simulink model "gait_player_right_leg"  (R2015b)
settings: Solver=FixedStepDiscrete  StartTime=0.0  StopTime=inf  FixedStep=.001  RelTol=1e-3
libraries: xpcethercatlib x19, slrtlib x7
settings Model: SimulationMode=external  Creator=rtheyyun  LastModifiedBy=tech
settings SolverCC: EnableConcurrentExecution=on  ConcurrentTasks=on
settings DataIOCC: SaveFinalState=on  SaveFormat=StructureWithTime  SignalLoggingSaveFormat=ModelDataLogs  InspectSignalLogs=on
settings OptimizationCC: BlockReduction=off  OptimizeBlockIOStorage=off  BufferReuse=off  GlobalBufferReuse=off  ExpressionFolding=off  ExpressionDepthLimit=2147483647  LocalBlockOutputs=off
settings DebuggingCC: ReadBeforeWriteMsg=DisableAll  WriteAfterWriteMsg=DisableAll  WriteAfterReadMsg=DisableAll  UnderspecifiedInitializationDetection=Classic  MergeDetectMultiDrivingBlocksExec=none  SolverPrmCheckMsg=warning  InheritedTsInSrcMsg=none  FcnCallInpInsideContextMsg=UseLocalSettings  StateNameClashWarn=warning
settings HardwareCC: ProdBitPerPointer=32  ProdLargestAtomicFloat=None  ProdWordSize=32  ProdLongLongMode=on  ProdHWDeviceType=Generic->32-bit x86 compatible
settings RTWCC: SystemTargetFile=slrt.tlc  TemplateMakefile=slrt_default_tmf  Description=Simulink Real-Time  RTWVerbose=off  RTWCompilerOptimization=on
settings SimulinkRealTimeCC: GeneratePreprocessorConditionals=Disable all  xPCisModelTimeout=off  xPCModelTimeoutSecs=20  xPCConcurrentTasks=on
settings ConfigComp: CovModelRefEnable=Off  CovSFcnEnable=off

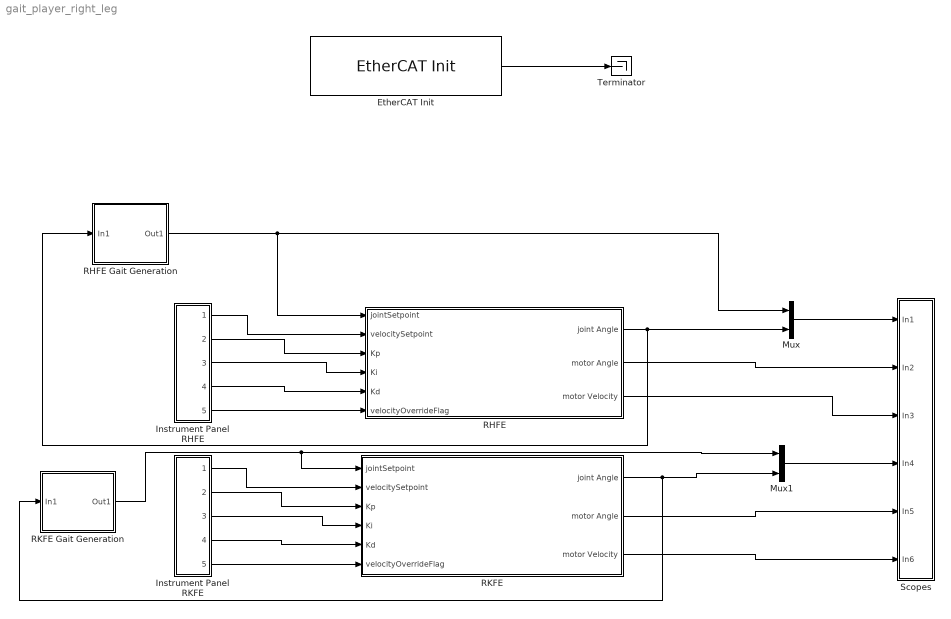
== system gait_player_right_leg ==
  "EtherCAT Init " : xpcethercatlib/EtherCAT Init   Priority=0  config_file=C:\Software\Simulink Realtime\Pre-recorded Gait\gait_player.xml  device_id=0  pci_bus=2  pci_slot=0  dctuning=0  enaDebug=off  enaDC=on  errLink=off  masterDbg=off  stateChgDbg=off  baseClock=off  masterCfg=off  logFile='c:\dbglog.txt'  sample_time=0.001000
  Instrument Panel RHFE : Subsystem
  Instrument Panel RKFE : Subsystem
  Mux : Mux  Inputs=2
  Mux1 : Mux  Inputs=2
  RHFE : Subsystem
  RHFE Gait Generation : Subsystem
  RKFE : Subsystem
  RKFE Gait Generation : Subsystem
  Scopes : Subsystem
  Terminator : Terminator
  wires:
  "EtherCAT Init "/1 -> Terminator/1
  Instrument Panel RHFE/1(Out2) -> RHFE/2("velocitySetpoint ")
  Instrument Panel RHFE/2(Out3) -> RHFE/3(Kp)
  Instrument Panel RHFE/3(Out4) -> RHFE/4(Ki)
  Instrument Panel RHFE/4(Out5) -> RHFE/5(Kd)
  Instrument Panel RHFE/5(Out6) -> RHFE/6(velocityOverrideFlag)
  Instrument Panel RKFE/1(Out2) -> RKFE/2("velocitySetpoint ")
  Instrument Panel RKFE/2(Out3) -> RKFE/3(Kp)
  Instrument Panel RKFE/3(Out4) -> RKFE/4(Ki)
  Instrument Panel RKFE/4(Out5) -> RKFE/5(Kd)
  Instrument Panel RKFE/5(Out6) -> RKFE/6(velocityOverrideFlag)
  RHFE/1(joint Angle) -> RHFE Gait Generation/1(In1), Mux/2
  RHFE/2(motor Angle) -> Scopes/2(In2)
  RHFE/3(motor Velocity) -> Scopes/3(In3)
  RKFE/1(joint Angle) -> RKFE Gait Generation/1(In1), Mux1/2
  RKFE/2(motor Angle) -> Scopes/5(In5)
  RKFE/3(motor Velocity) -> Scopes/6(In6)
  Mux/1 -> Scopes/1(In1)
  RHFE Gait Generation/1(Out1) -> RHFE/1(jointSetpoint), Mux/1
  Mux1/1 -> Scopes/4(In4)
  RKFE Gait Generation/1(Out1) -> RKFE/1(jointSetpoint), Mux1/1

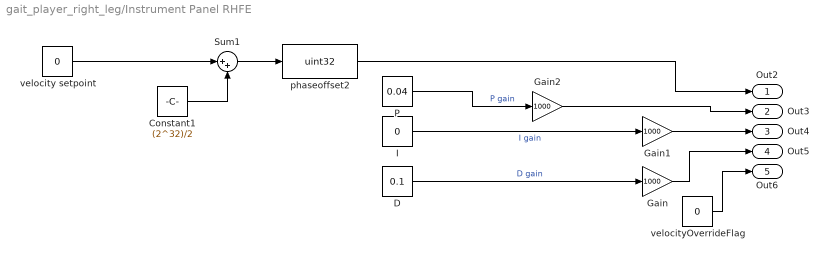
== system gait_player_right_leg/Instrument Panel RHFE ==
  Constant1 : Constant  Value=(2^32)/2
  D : Constant  Value=0.1  OutDataTypeStr=single
  Gain : Gain  Gain=1000  OutDataTypeStr=uint32
  Gain1 : Gain  Gain=1000  OutDataTypeStr=uint32
  Gain2 : Gain  Gain=1000  OutDataTypeStr=uint32
  I : Constant  Value=0  OutDataTypeStr=single
  P : Constant  Value=0.04  OutDataTypeStr=single
  Sum1 : Sum  Inputs=|++
  phaseoffset2 : DataTypeConversion  OutDataTypeStr=uint32
  velocity setpoint : Constant  Value=0  OutDataTypeStr=int16
  velocityOverrideFlag : Constant  Value=0  OutDataTypeStr=uint32
  Out2 : Outport
  Out3 : Outport  Port=2
  Out4 : Outport  Port=3
  Out5 : Outport  Port=4
  Out6 : Outport  Port=5
  wires:
  velocityOverrideFlag/1 -> Out6/1
  Gain2/1 -> Out3/1
  Constant1/1 -> Sum1/2
  Sum1/1 -> phaseoffset2/1
  velocity setpoint/1 -> Sum1/1
  phaseoffset2/1 -> Out2/1
  Gain1/1 -> Out4/1
  Gain/1 -> Out5/1
  I/1 -> Gain1/1  "I gain"
  D/1 -> Gain/1  "D gain"
  P/1 -> Gain2/1  "P gain"

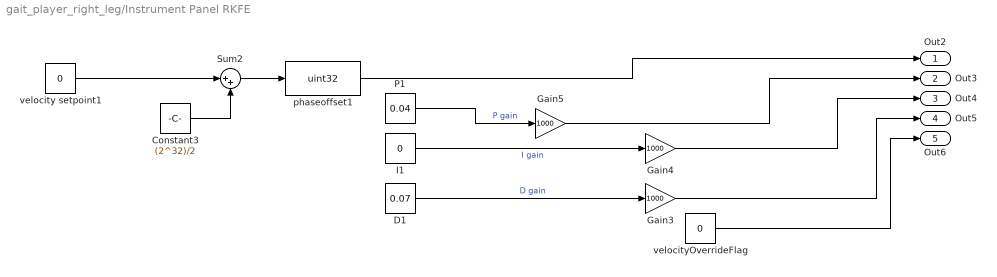
== system gait_player_right_leg/Instrument Panel RKFE ==
  Constant3 : Constant  Value=(2^32)/2
  D1 : Constant  Value=0.07  OutDataTypeStr=single
  Gain3 : Gain  Gain=1000  OutDataTypeStr=uint32
  Gain4 : Gain  Gain=1000  OutDataTypeStr=uint32
  Gain5 : Gain  Gain=1000  OutDataTypeStr=uint32
  I1 : Constant  Value=0  OutDataTypeStr=single
  P1 : Constant  Value=0.04  OutDataTypeStr=single
  Sum2 : Sum  Inputs=|++
  phaseoffset1 : DataTypeConversion  OutDataTypeStr=uint32
  velocity setpoint1 : Constant  Value=0  OutDataTypeStr=int16
  velocityOverrideFlag : Constant  Value=0  OutDataTypeStr=uint32
  Out2 : Outport
  Out3 : Outport  Port=2
  Out4 : Outport  Port=3
  Out5 : Outport  Port=4
  Out6 : Outport  Port=5
  wires:
  P1/1 -> Gain5/1  "P gain"
  Constant3/1 -> Sum2/2
  phaseoffset1/1 -> Out2/1
  Gain4/1 -> Out4/1
  Gain5/1 -> Out3/1
  I1/1 -> Gain4/1  "I gain"
  D1/1 -> Gain3/1  "D gain"
  Gain3/1 -> Out5/1
  velocityOverrideFlag/1 -> Out6/1
  velocity setpoint1/1 -> Sum2/1
  Sum2/1 -> phaseoffset1/1

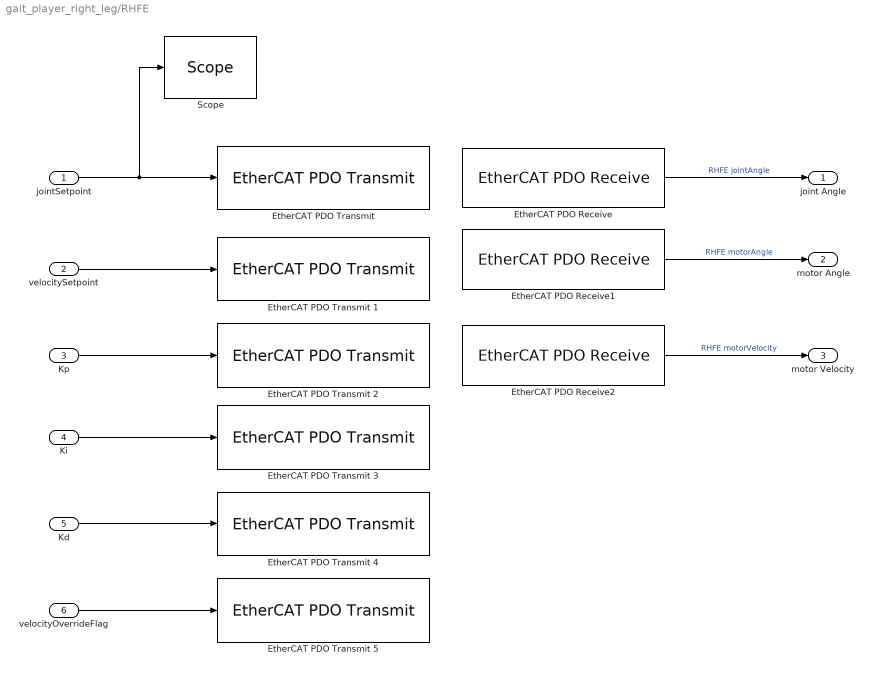
== system gait_player_right_leg/RHFE ==
  jointSetpoint : Inport
  "velocitySetpoint " : Inport  Port=2
  Kp : Inport  Port=3
  Ki : Inport  Port=4
  Kd : Inport  Port=5
  velocityOverrideFlag : Inport  Port=6
  EtherCAT PDO Receive : xpcethercatlib/EtherCAT PDO Receive  Priority=2  sig_name=RHFE.Inputs.jointAngle  sig_offset=208  sig_type=uint32  type_size=32  sig_dim=1  device_id=0  sample_time=0.001000
  EtherCAT PDO Receive1 : xpcethercatlib/EtherCAT PDO Receive  Priority=2  sig_name=RHFE.Inputs.motorAngle  sig_offset=240  sig_type=uint16  type_size=16  sig_dim=1  device_id=0  sample_time=0.001000
  EtherCAT PDO Receive2 : xpcethercatlib/EtherCAT PDO Receive  Priority=2  sig_name=RHFE.Inputs.motorVelocity  sig_offset=256  sig_type=int16  type_size=16  sig_dim=1  device_id=0  sample_time=0.001000
  "EtherCAT PDO Transmit " : xpcethercatlib/EtherCAT PDO Transmit   Priority=3  sig_name=RHFE.Outputs.jointSetpoint  sig_offset=208  sig_type=uint32  type_size=32  sig_dim=1  device_id=0  sample_time=0.001000
  EtherCAT PDO Transmit 1 : xpcethercatlib/EtherCAT PDO Transmit   Priority=3  sig_name=RHFE.Outputs.data0  sig_offset=240  sig_type=uint32  type_size=32  sig_dim=1  device_id=0  sample_time=0.001000
  EtherCAT PDO Transmit 2 : xpcethercatlib/EtherCAT PDO Transmit   Priority=3  sig_name=RHFE.Outputs.data1  sig_offset=272  sig_type=uint32  type_size=32  sig_dim=1  device_id=0  sample_time=0.001000
  EtherCAT PDO Transmit 3 : xpcethercatlib/EtherCAT PDO Transmit   Priority=3  sig_name=RHFE.Outputs.data2  sig_offset=304  sig_type=uint32  type_size=32  sig_dim=1  device_id=0  sample_time=0.001000
  EtherCAT PDO Transmit 4 : xpcethercatlib/EtherCAT PDO Transmit   Priority=3  sig_name=RHFE.Outputs.data3  sig_offset=336  sig_type=uint32  type_size=32  sig_dim=1  device_id=0  sample_time=0.001000
  EtherCAT PDO Transmit 5 : xpcethercatlib/EtherCAT PDO Transmit   Priority=3  sig_name=RHFE.Outputs.data4  sig_offset=368  sig_type=uint32  type_size=32  sig_dim=1  device_id=0  sample_time=0.001000
  "Scope " : slrtlib/Displays and Logging/Scope   scopeno=7  scopetype=Target  autostart=on  viewmode=Numerical  formatstr='%15.6f'  grid=on  ylimits=[0,0]  nosamples=3  noprepostsamples=0  interleave=1  triggermode=FreeRun  triggersignal=1  trigsignalfromport=off  triggerlevel=0.0  triggerslope=Either  triggerscope=1  triggersample=0  filename=data.dat  mode=Lazy  writesize=512  autorestart=off  dynamicfilemode=off  maxwritefilesize=512*1024^2
  joint Angle : Outport
  motor Angle : Outport  Port=2
  motor Velocity : Outport  Port=3
  wires:
  Ki/1 -> EtherCAT PDO Transmit 3/1
  Kd/1 -> EtherCAT PDO Transmit 4/1
  EtherCAT PDO Receive/1 -> joint Angle/1  "RHFE jointAngle"
  jointSetpoint/1 -> "Scope "/1, "EtherCAT PDO Transmit "/1
  "velocitySetpoint "/1 -> EtherCAT PDO Transmit 1/1
  EtherCAT PDO Receive2/1 -> motor Velocity/1  "RHFE motorVelocity"
  EtherCAT PDO Receive1/1 -> motor Angle/1  "RHFE motorAngle"
  velocityOverrideFlag/1 -> EtherCAT PDO Transmit 5/1
  Kp/1 -> EtherCAT PDO Transmit 2/1

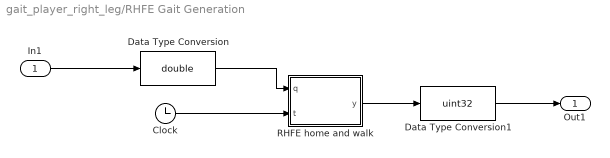
== system gait_player_right_leg/RHFE Gait Generation ==
  In1 : Inport
  Clock : Clock
  Data Type Conversion : DataTypeConversion  OutDataTypeStr=double
  Data Type Conversion1 : DataTypeConversion  OutDataTypeStr=uint32
  RHFE home and walk : MATLAB Function  TreatAsAtomicUnit=on
  Out1 : Outport
  wires:
  RHFE home and walk/1(y) -> Data Type Conversion1/1
  Data Type Conversion/1 -> RHFE home and walk/1(q)
  Data Type Conversion1/1 -> Out1/1
  Clock/1 -> RHFE home and walk/2(t)
  In1/1 -> Data Type Conversion/1

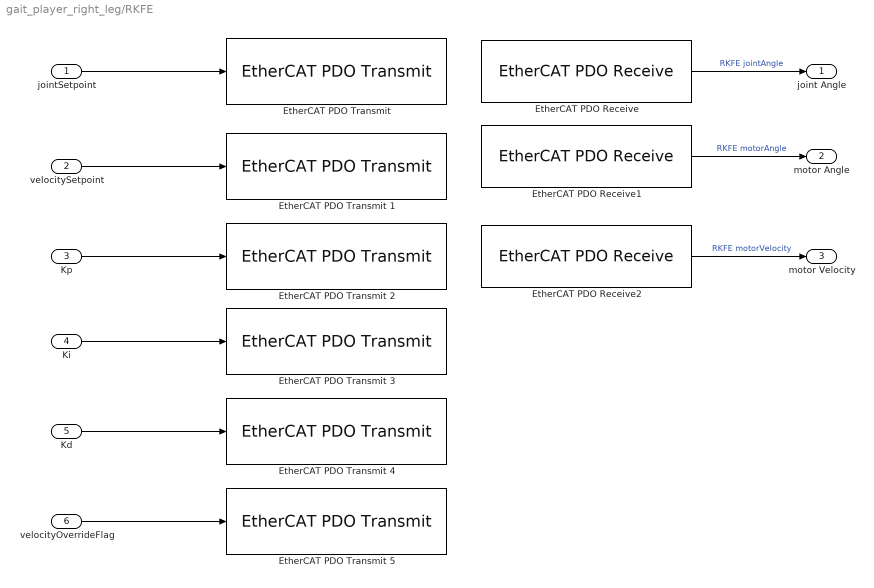
== system gait_player_right_leg/RKFE ==
  jointSetpoint : Inport
  "velocitySetpoint " : Inport  Port=2
  Kp : Inport  Port=3
  Ki : Inport  Port=4
  Kd : Inport  Port=5
  velocityOverrideFlag : Inport  Port=6
  EtherCAT PDO Receive : xpcethercatlib/EtherCAT PDO Receive  Priority=2  sig_name=RKFE.Inputs.jointAngle  sig_offset=496  sig_type=uint32  type_size=32  sig_dim=1  device_id=0  sample_time=0.001000
  EtherCAT PDO Receive1 : xpcethercatlib/EtherCAT PDO Receive  Priority=2  sig_name=RKFE.Inputs.motorAngle  sig_offset=528  sig_type=uint16  type_size=16  sig_dim=1  device_id=0  sample_time=0.001000
  EtherCAT PDO Receive2 : xpcethercatlib/EtherCAT PDO Receive  Priority=2  sig_name=RKFE.Inputs.motorVelocity  sig_offset=544  sig_type=int16  type_size=16  sig_dim=1  device_id=0  sample_time=0.001000
  "EtherCAT PDO Transmit " : xpcethercatlib/EtherCAT PDO Transmit   Priority=3  sig_name=RKFE.Outputs.jointSetpoint  sig_offset=496  sig_type=uint32  type_size=32  sig_dim=1  device_id=0  sample_time=0.001000
  EtherCAT PDO Transmit 1 : xpcethercatlib/EtherCAT PDO Transmit   Priority=3  sig_name=RKFE.Outputs.data0  sig_offset=528  sig_type=uint32  type_size=32  sig_dim=1  device_id=0  sample_time=0.001000
  EtherCAT PDO Transmit 2 : xpcethercatlib/EtherCAT PDO Transmit   Priority=3  sig_name=RKFE.Outputs.data1  sig_offset=560  sig_type=uint32  type_size=32  sig_dim=1  device_id=0  sample_time=0.001000
  EtherCAT PDO Transmit 3 : xpcethercatlib/EtherCAT PDO Transmit   Priority=3  sig_name=RKFE.Outputs.data2  sig_offset=592  sig_type=uint32  type_size=32  sig_dim=1  device_id=0  sample_time=0.001000
  EtherCAT PDO Transmit 4 : xpcethercatlib/EtherCAT PDO Transmit   Priority=3  sig_name=RKFE.Outputs.data3  sig_offset=624  sig_type=uint32  type_size=32  sig_dim=1  device_id=0  sample_time=0.001000
  EtherCAT PDO Transmit 5 : xpcethercatlib/EtherCAT PDO Transmit   Priority=3  sig_name=RKFE.Outputs.data4  sig_offset=656  sig_type=uint32  type_size=32  sig_dim=1  device_id=0  sample_time=0.001000
  joint Angle : Outport
  motor Angle : Outport  Port=2
  motor Velocity : Outport  Port=3
  wires:
  Ki/1 -> EtherCAT PDO Transmit 3/1
  Kd/1 -> EtherCAT PDO Transmit 4/1
  EtherCAT PDO Receive/1 -> joint Angle/1  "RKFE jointAngle"
  jointSetpoint/1 -> "EtherCAT PDO Transmit "/1
  "velocitySetpoint "/1 -> EtherCAT PDO Transmit 1/1
  EtherCAT PDO Receive2/1 -> motor Velocity/1  "RKFE motorVelocity"
  EtherCAT PDO Receive1/1 -> motor Angle/1  "RKFE motorAngle"
  velocityOverrideFlag/1 -> EtherCAT PDO Transmit 5/1
  Kp/1 -> EtherCAT PDO Transmit 2/1

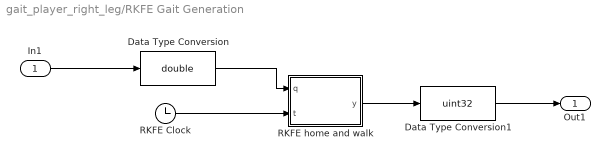
== system gait_player_right_leg/RKFE Gait Generation ==
  In1 : Inport
  Data Type Conversion : DataTypeConversion  OutDataTypeStr=double
  Data Type Conversion1 : DataTypeConversion  OutDataTypeStr=uint32
  RKFE Clock : Clock
  RKFE home and walk : MATLAB Function  TreatAsAtomicUnit=on
  Out1 : Outport
  wires:
  RKFE home and walk/1(y) -> Data Type Conversion1/1
  Data Type Conversion/1 -> RKFE home and walk/1(q)
  Data Type Conversion1/1 -> Out1/1
  RKFE Clock/1 -> RKFE home and walk/2(t)
  In1/1 -> Data Type Conversion/1

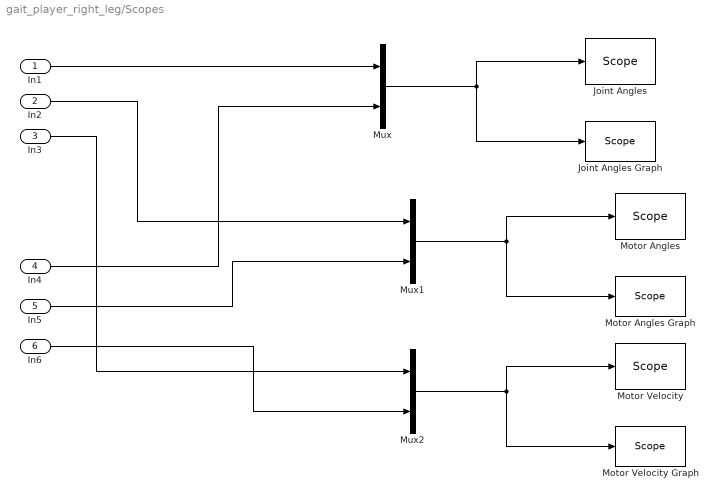
== system gait_player_right_leg/Scopes ==
  In1 : Inport
  In2 : Inport  Port=2
  In3 : Inport  Port=3
  In4 : Inport  Port=4
  In5 : Inport  Port=5
  In6 : Inport  Port=6
  Joint Angles : slrtlib/Displays and Logging/Scope   scopeno=1  scopetype=Target  autostart=on  viewmode=Numerical  formatstr='%15.6f'  grid=on  ylimits=[0,0]  nosamples=3  noprepostsamples=0  interleave=1  triggermode=FreeRun  triggersignal=1  trigsignalfromport=off  triggerlevel=0.0  triggerslope=Either  triggerscope=1  triggersample=0  filename=data.dat  mode=Lazy  writesize=512  autorestart=off  dynamicfilemode=off  maxwritefilesize=512*1024^2
  Joint Angles Graph : slrtlib/Displays and Logging/Scope   scopeno=4  scopetype=Target  autostart=on  viewmode=Graphical sliding  formatstr='%15.6f'  grid=on  ylimits=[0,0]  nosamples=10000  noprepostsamples=0  interleave=1  triggermode=FreeRun  triggersignal=1  trigsignalfromport=off  triggerlevel=0.0  triggerslope=Either  triggerscope=1  triggersample=0  filename=data.dat  mode=Lazy  writesize=512  autorestart=off  dynamicfilemode=off  maxwritefilesize=512*1024^2
  Motor Angles : slrtlib/Displays and Logging/Scope   scopeno=2  scopetype=Target  autostart=on  viewmode=Numerical  formatstr='%15.6f'  grid=on  ylimits=[0,0]  nosamples=3  noprepostsamples=0  interleave=1  triggermode=FreeRun  triggersignal=1  trigsignalfromport=off  triggerlevel=0.0  triggerslope=Either  triggerscope=1  triggersample=0  filename=data.dat  mode=Lazy  writesize=512  autorestart=off  dynamicfilemode=off  maxwritefilesize=512*1024^2
  Motor Angles Graph : slrtlib/Displays and Logging/Scope   scopeno=5  scopetype=Target  autostart=on  viewmode=Graphical sliding  formatstr='%15.6f'  grid=on  ylimits=[0,0]  nosamples=10000  noprepostsamples=0  interleave=1  triggermode=FreeRun  triggersignal=1  trigsignalfromport=off  triggerlevel=0.0  triggerslope=Either  triggerscope=1  triggersample=0  filename=data.dat  mode=Lazy  writesize=512  autorestart=off  dynamicfilemode=off  maxwritefilesize=512*1024^2
  Motor Velocity : slrtlib/Displays and Logging/Scope   scopeno=3  scopetype=Target  autostart=on  viewmode=Numerical  formatstr='%15.6f'  grid=on  ylimits=[0,0]  nosamples=3  noprepostsamples=0  interleave=1  triggermode=FreeRun  triggersignal=1  trigsignalfromport=off  triggerlevel=0.0  triggerslope=Either  triggerscope=1  triggersample=0  filename=data.dat  mode=Lazy  writesize=512  autorestart=off  dynamicfilemode=off  maxwritefilesize=512*1024^2
  Motor Velocity Graph : slrtlib/Displays and Logging/Scope   scopeno=6  scopetype=Target  autostart=on  viewmode=Graphical sliding  formatstr='%15.6f'  grid=on  ylimits=[0,0]  nosamples=10000  noprepostsamples=0  interleave=1  triggermode=FreeRun  triggersignal=1  trigsignalfromport=off  triggerlevel=0.0  triggerslope=Either  triggerscope=1  triggersample=0  filename=data.dat  mode=Lazy  writesize=512  autorestart=off  dynamicfilemode=off  maxwritefilesize=512*1024^2
  Mux : Mux  Inputs=2
  Mux1 : Mux  Inputs=2
  Mux2 : Mux  Inputs=2
  wires:
  Mux/1 -> Joint Angles Graph/1, Joint Angles/1
  In3/1 -> Mux2/1
  Mux2/1 -> Motor Velocity Graph/1, Motor Velocity/1
  In6/1 -> Mux2/2
  In4/1 -> Mux/2
  In1/1 -> Mux/1
  In5/1 -> Mux1/2
  In2/1 -> Mux1/1
  Mux1/1 -> Motor Angles Graph/1, Motor Angles/1

== matlab function gait_player_right_leg/RKFE Gait Generation/RKFE home and walk ==
  data: q input; y output; t input
function y  = fcn(q, t)
deadt = 0.2;
tf = 4;
persistent a;
bias = 350000;
if (q~=0)
    if (t > deadt)
        if (isempty(a))
            A = [1 0 0 0;1 tf tf^2 tf^3;0 1 0 0; 0 1 2*tf 3*tf^2];
            a = A\[q;bias;0;0];
        end
        
        if (t < tf+deadt)
            y = a(1)+a(2)*(t-deadt)+a(3)*(t-deadt)^2+a(4)*(t-deadt)^3;
        else
            y=30000*sin(pi/3*(t-tf-deadt))+bias;
        end
    else
        y = q;
    end
else
    y = q;
end

== matlab function gait_player_right_leg/RHFE Gait Generation/RHFE home and walk ==
  data: q input; y output; t input
function y  = fcn(q, t)
deadt = 0.4;
tf = 4;
persistent a;
bias = 380000;
if (q~=0)
    if (t > deadt)
        if (isempty(a))
            A = [1 0 0 0;1 tf tf^2 tf^3;0 1 0 0; 0 1 2*tf 3*tf^2];
            a = A\[q;bias;0;0];
        end
        
        if (t < tf+deadt)
            y = a(1)+a(2)*(t-deadt)+a(3)*(t-deadt)^2+a(4)*(t-deadt)^3;
        else
            y=30000*sin(pi/3*(t-tf-deadt))+bias;
        end
    else
        y = q;
    end
else
    y = q;
end
